simulink model "Regelstrecke"  (R2013b)
settings: Solver=ode45  StartTime=0.0  StopTime=10.0  RelTol=1e-3
values from neighbouring files (symbols this model uses):
  b1 = 2.39e6    (= 2390000)    [main3.m]
  c_oe = 36.5e6    (= 36500000)    [main3.m]
  c_p = 75e6    (= 75000000)    [main3.m]
  m_g = m_k + m_p    (= 268.7)    [main3.m]
settings Model: Creator=yjl_9  LastModifiedBy=yjl_9

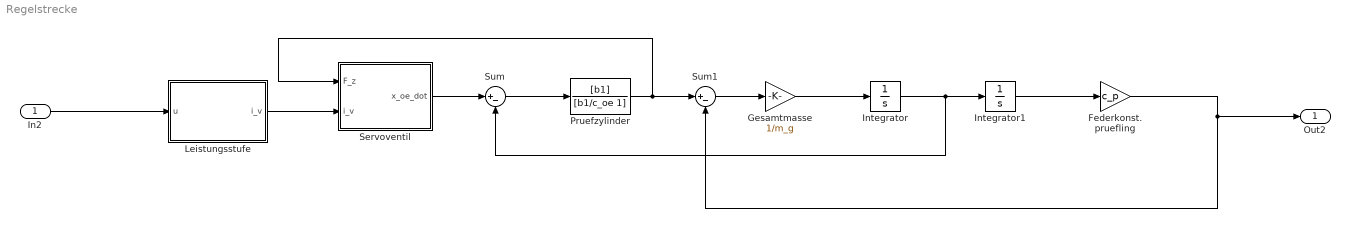
== system Regelstrecke ==
  In2 : Inport
  Federkonst. pruefling : Gain  Gain=c_p
  Gesamtmasse : Gain  Gain=1/m_g
  Integrator : Integrator
  Integrator1 : Integrator
  "Leistungsstufe " : MATLAB Function  TreatAsAtomicUnit=on
  Pruefzylinder : TransferFcn  Numerator=[b1]  Denominator=[b1/c_oe 1]
  "Servoventil " : MATLAB Function  TreatAsAtomicUnit=on
  Sum : Sum  Inputs=|+-
  Sum1 : Sum  Inputs=|+-
  Out2 : Outport
  wires:
  Federkonst. pruefling/1 -> Out2/1, Sum1/2
  "Leistungsstufe "/1(i_v) -> "Servoventil "/2(i_v)
  "Servoventil "/1(x_oe_dot) -> Sum/1
  Sum/1 -> Pruefzylinder/1
  Pruefzylinder/1 -> "Servoventil "/1(F_z), Sum1/1
  Sum1/1 -> Gesamtmasse/1
  Gesamtmasse/1 -> Integrator/1
  Integrator1/1 -> Federkonst. pruefling/1
  Integrator/1 -> Sum/2, Integrator1/1
  In2/1 -> "Leistungsstufe "/1(u)

== matlab function Regelstrecke/Servoventil  ==
  data: F_z input; i_v input; x_oe_dot output
function x_oe_dot = servoventil(F_z,i_v)
%#codegen
K_sv = 0.796; % [m/As]
F_N = 63000; % [N]
A = 1-(F_z/F_N)*sign(i_v);

if A > 0
    x_oe_dot = i_v*K_sv*sqrt(A);
else 
    x_oe_dot = 0;
end

== matlab function Regelstrecke/Leistungsstufe  ==
  data: u input; i_v output
function i_v  = leistungsstufe(u)
%codegen
i_max = 1; % [A]
K_L = 1; % [A/V]
    if u > 1
        i_v = i_max;
    elseif u < -1
        i_v = -i_max;
    else 
        i_v = K_L*u;
    end
